simulink subsystem "WindGFMTurbineInertia23a"  (R2023a)
settings: Solver=VariableStepAuto  StartTime=0.0  StopTime=10.0  RelTol=1e-3
model mask{Kp=0, D=0, H=0, KqI=0, Vd_ref=0, frequency=0, x_vir=0, r_vir=0, Imax=0, Radius1=0, pitch1=0, cp1=0, TSR1=0, airDensity1=0, wt1=0, rt1=0, Inertia1=0, p1=0, psim1=0, Ld1=0, Lq1=0, Rs1=0, Kp_dc_sm=0, Ki_dc_sm=0, Kpd=0, Kid=0, Kpq=0, Kiq=0}
  mask prompts: Kp "VSM frequency droop"; D "VSM damping"; H "VSM Inertia"; KqI "VSM Reactive power droop"; Vd_ref "Volatge Reference d-axis"; frequency "Reference frequency"; x_vir "Virtual reactance"; r_vir "Virtual resistance"; Imax "Current limit"; Radius1 "Radius of Turbine"; pitch1 "Pitch Angle Vector"; cp1 "Power Coefficient Table"; TSR1 "Tip Speed Ratio"; airDensity1 "Air Density"; wt1 "Wind Velocity Threshold"; rt1 "Rotational Velocity Threshold"; Inertia1 "Turbine Inertia"; p1 "Number of Pole Pairs"; psim1 "PM Flux Linkage"; Ld1 "Stator D-axis inductance (H)"; Lq1 "Stator Q-axis inductance (H)"; Rs1 "Stator Resistance (Ohms)"; Kp_dc_sm "Prportional Gain of Dc-link Controller"; Ki_dc_sm "Integral Gain of DC-link Controller"; Kpd "D-axis proportional Gain"; Kid "D-axis integral Gain"; Kpq "q-axis proportional Gain"; Kiq "q-axis integral Gain"
undefined symbols (not defined in the file): alpha, base, DiscIntNeverNeededParam, Ld, Lq, mpptPower, mpptWindSpeed, p, psim, Rs, Ts, windController, windInverter, windTurbine
libraries: nesl_utility x14, ee_lib x9, fl_lib x7, slpidlib x5, eeTransforms x5, eeGeneralControl x2, simulink x2, eePowerMeasurement x1, eePmsmCurrentController x1
(part 1 of 2)
settings Model: Creator=rajarshd  LastModifiedBy=rajarshd
settings DebuggingCC: SubsystemReferenceDiagnosticForUnitTest=warning

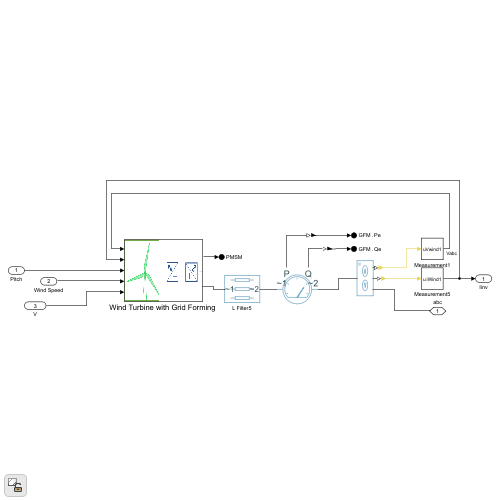
[thumbnail: Simulink's stored preview of the top-level diagram]
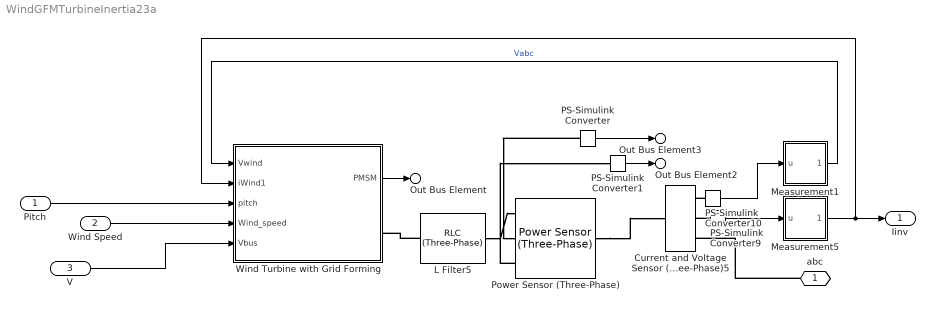
== system WindGFMTurbineInertia23a ==
  Pitch : Inport
  Wind Speed : Inport  Port=2
  V : Inport  Port=3
  Current and Voltage Sensor (Three-Phase)5 : ee_lib/Sensors & Transducers/Current and Voltage Sensor (Three-Phase)  vMeasurementType=ee.enum.vmeasurement.lg  outputUnit=ee.enum.unit.pu  SRated=base.mVA A*V  VRated=base.kV V  I_specify=off  I_priority=None  I=[0, 0, 0] A  I_nominal_specify=off  I_nominal_unit=A  I_nominal_value=1  V_specify=off  V_priority=None  V=[0, 0, 0] V  V_nominal_specify=off  V_nominal_unit=V  V_nominal_value=1
      settings: InternalSimscapePortConfiguration="{\"Bottom\":[],\"Left\":[{\"id\":\"N1\",\"label\":\"~1\",\"type\":\"foundation.electrical.three_phase\"}],\"Right\":[{\"id\":\"V_output\",\"label\":\"V\",\"type\":\"output\"},{\"id\":\"I_output\",\"label\":\"I\",\"type\":\"output\"},{\"id\":\"N2\",\"label\":\"~2\",\"type\":\"foundation.electrical.three_phase\"}],\"Top\":[]}"
  L Filter5 : ee_lib/Passive/RLC Assemblies/RLC (Three-Phase)  component_structure=ee.enum.rlc.structure.L  R=1e-3 Ohm  L=windInverter.l*1 H  C=1e-6 F  R_parasitic=0 Ohm  G_parasitic=0 1/Ohm  IL_specify=off  IL_priority=High  IL=[0, 0, 0] A  IL_nominal_specify=off  IL_nominal_unit=A  IL_nominal_value=1  VC_specify=off  VC_priority=High  VC=[0, 0, 0] V  VC_nominal_specify=off  VC_nominal_unit=V  VC_nominal_value=1
      settings: InternalSimscapePortConfiguration="{\"Bottom\":[],\"Left\":[{\"id\":\"N1\",\"label\":\"~1\",\"type\":\"foundation.electrical.three_phase\"}],\"Right\":[{\"id\":\"N2\",\"label\":\"~2\",\"type\":\"foundation.electrical.three_phase\"}],\"Top\":[]}"
  Measurement1 : Subsystem
  Measurement5 : Subsystem
  PS-Simulink Converter{,1,9..10} (4 alike) : nesl_utility/PS-Simulink Converter  PhysicalDomain=network_engine_domain  SubClassName=ps_output  LeftPortType=input  RightPortType=output  PseudoPeriodic=off  Frequencies=[]  VectorFormat=inherit  Unit=inherit  AffineConversion=off
  Power Sensor (Three-Phase) : ee_lib/Sensors & Transducers/Power Sensor (Three-Phase)  load_type=ee.enum.passive.type_balanced.balanced  f0=60 Hz  config=ee.enum.with_neutral.no  rho=1
      settings: InternalSimscapePortConfiguration="{\"Bottom\":[],\"Left\":[{\"id\":\"N1\",\"label\":\"~1\",\"type\":\"foundation.electrical.three_phase\"}],\"Right\":[{\"id\":\"N2\",\"label\":\"~2\",\"type\":\"foundation.electrical.three_phase\"}],\"Top\":[{\"id\":\"Pm\",\"label\":\"P\",\"type\":\"output\"},{\"id\":\"Qm\",\"label\":\"Q\",\"type\":\"output\"}]}"
  "Wind Turbine with Grid Forming " : Subsystem
      mask Display: image('T4wind.png'); % Use "Edit Image" on toolstrip to change.
  abc : PMIOPort  Side=Right
  Iinv : Outport
  Out Bus Element : Outport  Port=2  PortName=PMSM
  Out Bus Element2 : Outport  Port=3  PortName=GFM  Element=Qe
  Out Bus Element3 : Outport  Port=3  PortName=GFM  Element=Pe
  wires:
  V/1 -> "Wind Turbine with Grid Forming "/5(Vbus)
  Measurement1/1(Vwind1) -> "Wind Turbine with Grid Forming "/1(Vwind)  "Vabc"
  PS-Simulink Converter9/1 -> Measurement5/1(u)
  Measurement5/1(iWind1) -> "Wind Turbine with Grid Forming "/2(iWind1), Iinv/1
  PS-Simulink Converter10/1 -> Measurement1/1(u)
  Wind Speed/1 -> "Wind Turbine with Grid Forming "/4(Wind_speed)
  Pitch/1 -> "Wind Turbine with Grid Forming "/3(pitch)
  "Wind Turbine with Grid Forming "/1(PMSM) -> Out Bus Element/1
  PS-Simulink Converter/1 -> Out Bus Element3/1
  PS-Simulink Converter1/1 -> Out Bus Element2/1
  connections:
  L Filter5/LConn1 -- "Wind Turbine with Grid Forming "/RConn1
  PS-Simulink Converter9/LConn1 -- Current and Voltage Sensor (Three-Phase)5/RConn2
  PS-Simulink Converter10/LConn1 -- Current and Voltage Sensor (Three-Phase)5/RConn1
  abc/RConn1 -- Current and Voltage Sensor (Three-Phase)5/RConn3
  Power Sensor (Three-Phase)/RConn1 -- Current and Voltage Sensor (Three-Phase)5/LConn1
  PS-Simulink Converter/LConn1 -- Power Sensor (Three-Phase)/LConn2
  Power Sensor (Three-Phase)/LConn3 -- PS-Simulink Converter1/LConn1
  L Filter5/RConn1 -- Power Sensor (Three-Phase)/LConn1

== system WindGFMTurbineInertia23a/Measurement1 ==
  u : Inport
  Lead-Lag (Discrete or Continuous) : eeGeneralControl/Lead-Lag (Discrete or Continuous)  T1=0  T2=windController.tSensor  B=inf  A=-inf  init_option=Inherited from block input  x0=0  Ts=Ts
      settings: LibrarySourceBlock=|
      | ee_sl_lib/General Control/Lead-Lag
      | (Discrete or Continuous)
  Out Bus Element : Outport  PortName=Vwind1
  wires:
  u/1 -> Lead-Lag (Discrete or Continuous)/1
  Lead-Lag (Discrete or Continuous)/1 -> Out Bus Element/1

== system WindGFMTurbineInertia23a/Measurement5 ==
  u : Inport
  Lead-Lag (Discrete or Continuous) : eeGeneralControl/Lead-Lag (Discrete or Continuous)  T1=0  T2=windController.tSensor  B=inf  A=-inf  init_option=Inherited from block input  x0=0  Ts=Ts
      settings: LibrarySourceBlock=|
      | ee_sl_lib/General Control/Lead-Lag
      | (Discrete or Continuous)
  Out Bus Element : Outport  PortName=iWind1  Element=1
  wires:
  u/1 -> Lead-Lag (Discrete or Continuous)/1
  Lead-Lag (Discrete or Continuous)/1 -> Out Bus Element/1

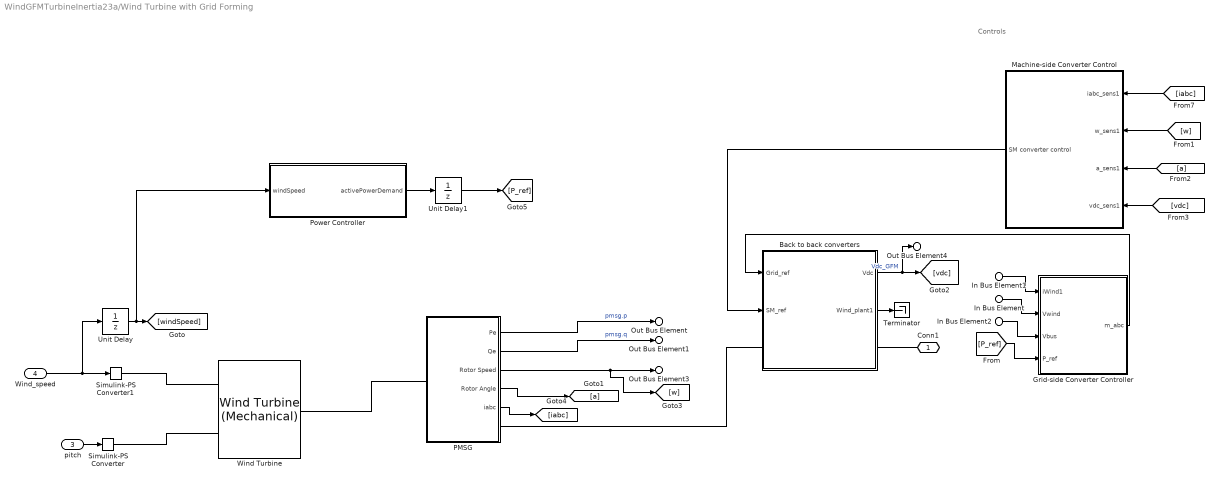
== system WindGFMTurbineInertia23a/Wind Turbine with Grid Forming  ==
  note: Controls
  In Bus Element : Inport  PortName=Vwind
  In Bus Element1 : Inport  Port=2  PortName=iWind1
  pitch : Inport  Port=3
  Wind_speed : Inport  Port=4
  In Bus Element2 : Inport  Port=5  PortName=Vbus
  " Grid-side Converter Controller" : Subsystem
  Back to back converters : Subsystem
  Machine-side Converter Control : Subsystem
  PMSG : Subsystem
  Power Controller : Subsystem
  Simulink-PS Converter : nesl_utility/Simulink-PS Converter  PhysicalDomain=network_engine_domain  SubClassName=ps_input  LeftPortType=input  RightPortType=output  PseudoPeriodic=off  Frequencies=[]  NoiseDistribution=none  NoiseParameters=[]  Unit=1  AffineConversion=off  FilteringAndDerivatives=provide  SimscapeFilterOrder=1  InputFilterTimeConstant=0.001  UdotUserProvided=0
  Simulink-PS Converter1 : nesl_utility/Simulink-PS Converter  PhysicalDomain=network_engine_domain  SubClassName=ps_input  LeftPortType=input  RightPortType=output  PseudoPeriodic=off  Frequencies=[]  NoiseDistribution=none  NoiseParameters=[]  Unit=1  AffineConversion=off  FilteringAndDerivatives=provide  SimscapeFilterOrder=1  InputFilterTimeConstant=0.001  UdotUserProvided=0
  Terminator : Terminator
  Unit Delay : UnitDelay  SampleTime=-1  HasFrameUpgradeWarning=on
  Unit Delay1 : UnitDelay  SampleTime=-1  HasFrameUpgradeWarning=on
  "Wind Turbine " : ee_lib/Electromechanical/Wind Turbine (Mechanical)  R_rotor=Radius1 m  pitch_TLU=pitch1 deg  lambda_TLU=TSR1  Cp_TLU=cp1  v_thr=wt1 m/s  w_thr=rt1 rad/s  rho_air=airDensity1 kg/m^3  includeInertia=true  J=Inertia1 kg*m^2  lam=1 N*m*s/rad  w_specify=on  w_priority=Low  w=2.26*2 rad/s  w_nominal_specify=off  w_nominal_unit=rad/s  w_nominal_value=1  t_specify=off  t_priority=None  t=0 N*m  t_nominal_specify=off  t_nominal_unit=N*m  t_nominal_value=1  Torque_specify=off  Torque_priority=None  Torque=0 N*m  Torque_nominal_specify=off  Torque_nominal_unit=N*m  Torque_nominal_value=1
      settings: InternalSimscapePortConfiguration="{\"Bottom\":[],\"Left\":[{\"id\":\"vWind\",\"label\":\"V\",\"type\":\"input\"},{\"id\":\"pitch\",\"label\":\"β\",\"type\":\"input\"}],\"Right\":[{\"id\":\"R\",\"label\":\"R\",\"type\":\"foundation.mechanical.rotational.rotational\"}],\"Top\":[]}"
  Conn1 : PMIOPort  Side=Right
  Out Bus Element : Outport  PortName=PMSM  Element=P_GFM
  Out Bus Element1 : Outport  PortName=PMSM  Element=Q_GFM
  Out Bus Element3 : Outport  PortName=PMSM  Element=w_speed_GFM
  Out Bus Element4 : Outport  PortName=PMSM  Element=Vdc_GFM
  wires:
  [iabc] -> Machine-side Converter Control/1(iabc_sens1)
  [w] -> Machine-side Converter Control/2(w_sens1)
  [a] -> Machine-side Converter Control/3(a_sens1)
  [vdc] -> Machine-side Converter Control/4(vdc_sens1)
  PMSG/3(Rotor Speed) -> [w], Out Bus Element3/1
  PMSG/2(Qe) -> Out Bus Element1/1  "pmsg.q"
  In Bus Element1/1 -> " Grid-side Converter Controller"/1(iWind1)
  Wind_speed/1 -> Simulink-PS Converter1/1, Unit Delay/1
  pitch/1 -> Simulink-PS Converter/1
  PMSG/5(iabc) -> [iabc]
  Back to back converters/1(Vdc) -> Out Bus Element4/1, [vdc]  "Vdc_GFM"
  PMSG/4(Rotor Angle) -> [a]
  PMSG/1(Pe) -> Out Bus Element/1  "pmsg.p"
  Unit Delay/1 -> Power Controller/1(windSpeed), [windSpeed]
  In Bus Element/1 -> " Grid-side Converter Controller"/2(Vwind)
  In Bus Element2/1 -> " Grid-side Converter Controller"/3(Vbus)
  Unit Delay1/1 -> [P_ref]
  Power Controller/1(activePowerDemand) -> Unit Delay1/1
  [P_ref] -> " Grid-side Converter Controller"/4(P_ref)
  Back to back converters/2(Wind_plant1) -> Terminator/1
  Machine-side Converter Control/1(SM converter control) -> Back to back converters/2(SM_ref)
  " Grid-side Converter Controller"/1(m_abc) -> Back to back converters/1(Grid_ref)
  connections:
  PMSG/RConn1 -- Back to back converters/LConn1
  "Wind Turbine "/RConn1 -- PMSG/LConn1
  "Wind Turbine "/LConn2 -- Simulink-PS Converter/RConn1
  "Wind Turbine "/LConn1 -- Simulink-PS Converter1/RConn1
  Conn1/RConn1 -- Back to back converters/RConn1

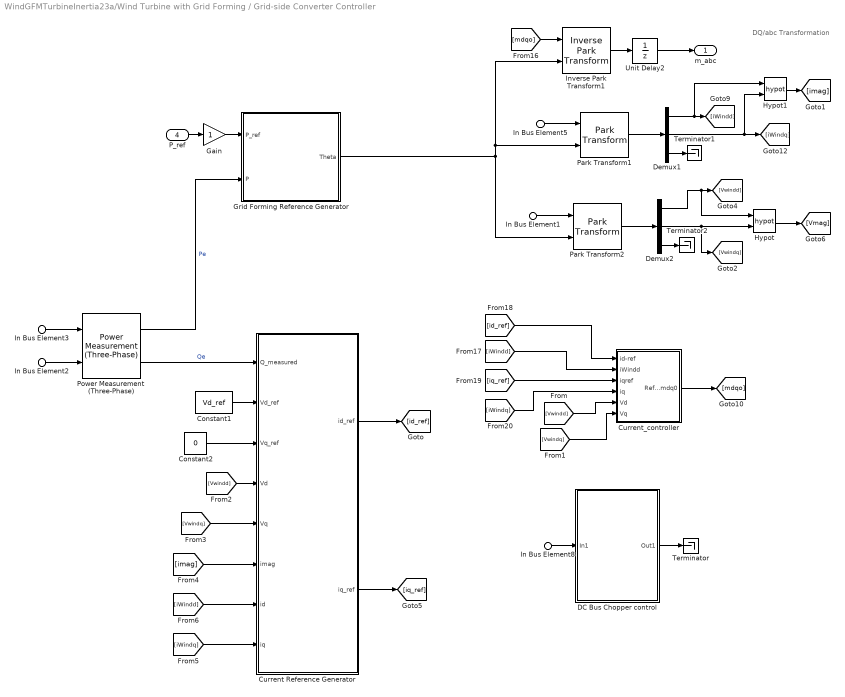
== system WindGFMTurbineInertia23a/Wind Turbine with Grid Forming / Grid-side Converter Controller ==
  note: DQ/abc Transformation
  In Bus Element5 : Inport  PortName=iWind1
  In Bus Element2 : Inport  PortName=iWind1
  In Bus Element1 : Inport  Port=2  PortName=Vwind
  In Bus Element3 : Inport  Port=2  PortName=Vwind
  In Bus Element8 : Inport  Port=3  PortName=Vbus  Element=Vmag
  P_ref : Inport  Port=4
  Constant1 : Constant  Value=Vd_ref
  Constant2 : Constant  Value=0
  Current Reference Generator : Subsystem
  Current_controller : Subsystem
  "DC Bus Chopper control " : Subsystem
  Demux1 : Demux  Outputs=3
  Demux2 : Demux  Outputs=3
  Gain : Gain
  Grid Forming Reference Generator : Subsystem
  Hypot : Math  Operator=hypot  SignedPower=on  RndMeth=Zero
  Hypot1 : Math  Operator=hypot
  Inverse Park Transform1 : eeTransforms/Inverse Park Transform  AxisAlignment=Q-axis  PowerInvariant=off
  Park Transform1 : eeTransforms/Park Transform  AxisAlignment=Q-axis  PowerInvariant=off
  Park Transform2 : eeTransforms/Park Transform  AxisAlignment=Q-axis  PowerInvariant=off
  Power Measurement (Three-Phase) : eePowerMeasurement/Power Measurement (Three-Phase)  LabelModeActiveChoice=Discrete  F=60  K=[1]  Seq=Positive  Ts=Ts
  Terminator : Terminator
  Terminator1 : Terminator
  Terminator2 : Terminator
  Unit Delay2 : UnitDelay  SampleTime=Ts  HasFrameUpgradeWarning=on
  m_abc : Outport
  wires:
  Gain/1 -> Grid Forming Reference Generator/1(P_ref)
  "DC Bus Chopper control "/1(Out1) -> Terminator/1
  In Bus Element8/1 -> "DC Bus Chopper control "/1(In1)
  [iWindq] -> Current Reference Generator/8(iq)
  [iWindd] -> Current Reference Generator/7(id)
  [imag] -> Current Reference Generator/6(imag)
  Hypot1/1 -> [imag]
  [Vwindq] -> Current Reference Generator/5(Vq)
  [Vwindd] -> Current Reference Generator/4(Vd)
  Constant2/1 -> Current Reference Generator/3(Vq_ref)
  Constant1/1 -> Current Reference Generator/2(Vd_ref)
  Power Measurement (Three-Phase)/2 -> Current Reference Generator/1(Q_measured)  "Qe"
  Power Measurement (Three-Phase)/1 -> Grid Forming Reference Generator/2(P)  "Pe"
  Current Reference Generator/2(iq_ref) -> [iq_ref]
  Current Reference Generator/1(id_ref) -> [id_ref]
  Grid Forming Reference Generator/1(Theta) -> Park Transform2/2, Park Transform1/2, Inverse Park Transform1/2
  In Bus Element3/1 -> Power Measurement (Three-Phase)/1
  In Bus Element2/1 -> Power Measurement (Three-Phase)/2
  Hypot/1 -> [Vmag]
  [Vwindq] -> Current_controller/6(Vq)
  [Vwindd] -> Current_controller/5(Vd)
  In Bus Element1/1 -> Park Transform2/1
  Demux2/2 -> [Vwindq], Hypot/2
  Demux2/3 -> Terminator2/1
  Demux2/1 -> [Vwindd], Hypot/1
  Park Transform2/1 -> Demux2/1
  Current_controller/1(Refrence_mdq0) -> [mdqo]
  Inverse Park Transform1/1 -> Unit Delay2/1
  Demux1/2 -> [iWindq], Hypot1/2
  Unit Delay2/1 -> m_abc/1
  Demux1/1 -> [iWindd], Hypot1/1
  Demux1/3 -> Terminator1/1
  [mdqo] -> Inverse Park Transform1/1
  Park Transform1/1 -> Demux1/1
  [id_ref] -> Current_controller/1(id-ref)
  [iq_ref] -> Current_controller/3(iqref)
  [iWindq] -> Current_controller/4(iq)
  [iWindd] -> Current_controller/2(iWindd)
  In Bus Element5/1 -> Park Transform1/1
  P_ref/1 -> Gain/1

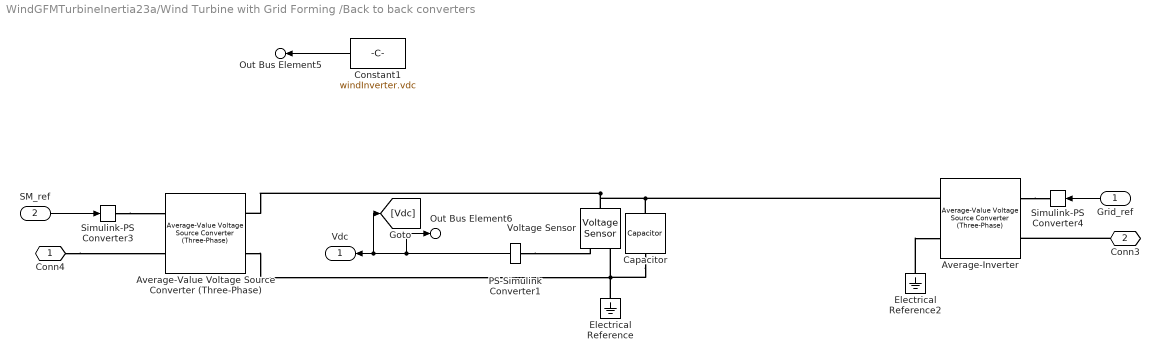
== system WindGFMTurbineInertia23a/Wind Turbine with Grid Forming /Back to back converters ==
  Grid_ref : Inport
  SM_ref : Inport  Port=2
  Average-Inverter : ee_lib/Semiconductors & Converters/Converters/Average-Value Voltage Source Converter (Three-Phase)  port_option=ee.enum.threePhasePort.composite  frequency_option=ee.enum.converters.frequency.variable  FRated=60 Hz  losses_parameterization=ee.enum.converters.losses.fixed  Pfixed=1 W  ks=0.01  kc1=1.7 V  kc2=0.01 Ohm  Ploss_vect=[100, 800, 1870, 3250, 4900] W  Irms_vect=[10, 100, 200, 300, 400] A  Vdc_nom=300 V  thermal_mass=30000 J/K  temperature_specify=off  temperature_priority=High  temperature=298.15 K  temperature_nominal_specify=off  temperature_nominal_unit=K  temperature_nominal_value=1
      settings: InternalSimscapePortConfiguration="{\"Bottom\":[],\"Left\":[{\"id\":\"ModWave\",\"label\":\"ModWave\",\"type\":\"input\"},{\"id\":\"N\",\"label\":\"~\",\"type\":\"foundation.electrical.three_phase\"}],\"Right\":[{\"id\":\"p\",\"label\":\"+\",\"type\":\"foundation.electrical.electrical\"},{\"id\":\"n\",\"label\":\"-\",\"type\":\"foundation.electrical.electrical\"}],\"Top\":[]}"
  Average-Value Voltage Source Converter (Three-Phase) : ee_lib/Semiconductors & Converters/Converters/Average-Value Voltage Source Converter (Three-Phase)  port_option=ee.enum.threePhasePort.composite  frequency_option=ee.enum.converters.frequency.variable  FRated=60 Hz  losses_parameterization=ee.enum.converters.losses.fixed  Pfixed=1 W  ks=0.01  kc1=1.7 V  kc2=0.01 Ohm  Ploss_vect=[100, 800, 1870, 3250, 4900] W  Irms_vect=[10, 100, 200, 300, 400] A  Vdc_nom=300 V  thermal_mass=30000 J/K  temperature_specify=off  temperature_priority=High  temperature=298.15 K  temperature_nominal_specify=off  temperature_nominal_unit=K  temperature_nominal_value=1
      settings: InternalSimscapePortConfiguration="{\"Bottom\":[],\"Left\":[{\"id\":\"ModWave\",\"label\":\"ModWave\",\"type\":\"input\"},{\"id\":\"N\",\"label\":\"~\",\"type\":\"foundation.electrical.three_phase\"}],\"Right\":[{\"id\":\"p\",\"label\":\"+\",\"type\":\"foundation.electrical.electrical\"},{\"id\":\"n\",\"label\":\"-\",\"type\":\"foundation.electrical.electrical\"}],\"Top\":[]}"
  Capacitor : fl_lib/Electrical/Electrical Elements/Capacitor  c=windInverter.c*2.5 F  r=0.001 Ohm  g=0 1/Ohm  i_specify=off  i_priority=None  i=0 A  i_nominal_specify=off  i_nominal_unit=A  i_nominal_value=1  v_specify=off  v_priority=None  v=0 V  v_nominal_specify=off  v_nominal_unit=V  v_nominal_value=1  vc_specify=on  vc_priority=None  vc=windInverter.vdc V  vc_nominal_specify=off  vc_nominal_unit=V  vc_nominal_value=1
  Constant1 : Constant  Value=windInverter.vdc  SampleTime=Ts
  Electrical Reference : fl_lib/Electrical/Electrical Elements/Electrical Reference
  Electrical Reference2 : fl_lib/Electrical/Electrical Elements/Electrical Reference
  PS-Simulink Converter1 : nesl_utility/PS-Simulink Converter  PhysicalDomain=network_engine_domain  SubClassName=ps_output  LeftPortType=input  RightPortType=output  PseudoPeriodic=off  Frequencies=[]  VectorFormat=inherit  Unit=V  AffineConversion=off
  Simulink-PS Converter3 : nesl_utility/Simulink-PS Converter  PhysicalDomain=network_engine_domain  SubClassName=ps_input  LeftPortType=input  RightPortType=output  PseudoPeriodic=off  Frequencies=[]  NoiseDistribution=none  NoiseParameters=[]  Unit=1  AffineConversion=off  FilteringAndDerivatives=provide  SimscapeFilterOrder=1  InputFilterTimeConstant=0.001  UdotUserProvided=0
  Simulink-PS Converter4 : nesl_utility/Simulink-PS Converter  PhysicalDomain=network_engine_domain  SubClassName=ps_input  LeftPortType=input  RightPortType=output  PseudoPeriodic=off  Frequencies=[]  NoiseDistribution=none  NoiseParameters=[]  Unit=1  AffineConversion=off  FilteringAndDerivatives=provide  SimscapeFilterOrder=1  InputFilterTimeConstant=0.001  UdotUserProvided=0
  Voltage Sensor : fl_lib/Electrical/Electrical Sensors/Voltage Sensor
  Conn4 : PMIOPort  Side=Left
  Conn3 : PMIOPort  Port=2  Side=Right
  Vdc : Outport
  Out Bus Element6 : Outport  Port=2  PortName=Wind_plant1  Element=Vdc_measured
  Out Bus Element5 : Outport  Port=2  PortName=Wind_plant1  Element=windInverter.vdc
  wires:
  PS-Simulink Converter1/1 -> Out Bus Element6/1, Vdc/1, [Vdc]
  Grid_ref/1 -> Simulink-PS Converter4/1
  SM_ref/1 -> Simulink-PS Converter3/1
  Constant1/1 -> Out Bus Element5/1
  connections:
  Capacitor/LConn1 -- Voltage Sensor/LConn1 -- Average-Value Voltage Source Converter (Three-Phase)/RConn1 -- Average-Inverter/RConn1
  Capacitor/RConn1 -- Voltage Sensor/RConn2 -- Average-Value Voltage Source Converter (Three-Phase)/RConn2 -- Electrical Reference/LConn1
  PS-Simulink Converter1/LConn1 -- Voltage Sensor/RConn1
  Electrical Reference2/LConn1 -- Average-Inverter/RConn2
  Conn4/RConn1 -- Average-Value Voltage Source Converter (Three-Phase)/LConn2
  Average-Inverter/LConn1 -- Simulink-PS Converter4/RConn1
  Simulink-PS Converter3/RConn1 -- Average-Value Voltage Source Converter (Three-Phase)/LConn1
  Conn3/RConn1 -- Average-Inverter/LConn2

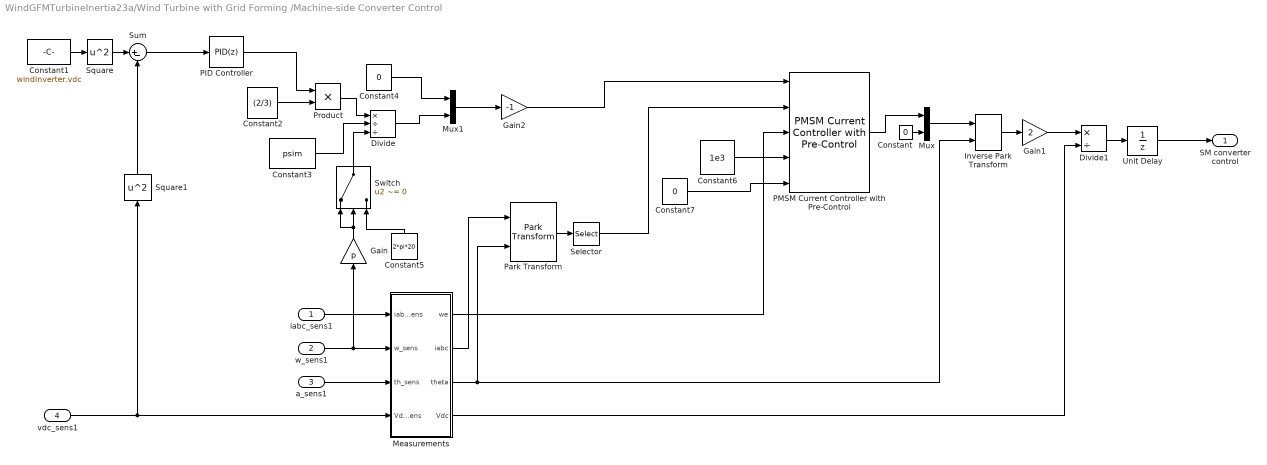
== system WindGFMTurbineInertia23a/Wind Turbine with Grid Forming /Machine-side Converter Control ==
  iabc_sens1 : Inport
  w_sens1 : Inport  Port=2
  a_sens1 : Inport  Port=3
  vdc_sens1 : Inport  Port=4
  Constant : Constant  Value=0  SampleTime=-1
  Constant1 : Constant  Value=windInverter.vdc
  Constant2 : Constant  Value=(2/3)
  Constant3 : Constant  Value=psim
  Constant4 : Constant  Value=0
  Constant5 : Constant  Value=2*pi*20
  Constant6 : Constant  Value=1e3  VectorParams1D=off  SampleTime=-1
  Constant7 : Constant  Value=0
  Divide : Product  Inputs=*//
  Divide1 : Product  Inputs=*/
  Gain : Gain  Gain=p
  Gain1 : Gain  Gain=2
  Gain2 : Gain  Gain=-1
  Inverse Park Transform : eeTransforms/Inverse Park Transform  AxisAlignment=Q-axis  PowerInvariant=off
  Measurements : Subsystem
  Mux : Mux  Inputs=2
  Mux1 : Mux  Inputs=2
  PID Controller : slpidlib/PID Controller  Controller=PID  Form=Parallel  TimeDomain=Discrete-time  UseExternalTs=off  SampleTime=-1  IntegratorMethod=Forward Euler  FilterMethod=Forward Euler  ControllerParametersSource=internal  P=Kp_dc_sm  I=Ki_dc_sm  UseKiTs=off  D=0  N=100  UseFilter=on  TunerSelectOption=Transfer Function Based (PID Tuner App)  InitialConditionSource=internal  InitialConditionForIntegrator=0  InitialConditionForFilter=0  DifferentiatorICPrevScaledInput=0  ExternalReset=none  TrackingMode=off  Kt=1  LimitOutput=off  SatLimitsSource=internal  UpperSaturationLimit=10e6  LowerSaturationLimit=-10e6  LinearizeAsGain=on  AntiWindupMode=none  Kb=1  LimitIntegrator=off  UpperIntegratorSaturationLimit=inf  LowerIntegratorSaturationLimit=-inf  POutMin=[]  POutMax=[]  IOutMin=[]  IOutMax=[]  DOutMin=[]  DOutMax=[]  NOutMin=[]  NOutMax=[]  SumOutMin=[]  SumOutMax=[]  SaturationOutMin=[]  SaturationOutMax=[]  PParamMin=[]  PParamMax=[]  IParamMin=[]  IParamMax=[]  DParamMin=[]  DParamMax=[]  NParamMin=[]  NParamMax=[]  KbParamMin=[]  KbParamMax=[]  KtParamMin=[]  KtParamMax=[]  KbOutMin=[]  KbOutMax=[]  KtOutMin=[]  KtOutMax=[]  IntegratorOutMin=[]  IntegratorOutMax=[]  FilterOutMin=[]  FilterOutMax=[]  SumI1OutMin=[]  SumI1OutMax=[]  SumI2OutMin=[]  SumI2OutMax=[]  SumI3OutMin=[]  SumI3OutMax=[]  SumI4OutMin=[]  SumI4OutMax=[]  SumDOutMin=[]  SumDOutMax=[]  DifferentiatorOutMin=[]  DifferentiatorOutMax=[]  FilterDiffOutCoefMin=[]  FilterDiffOutCoefMax=[]  ReciprocalOutMin=[]  ReciprocalOutMax=[]  SumDenOutMin=[]  SumDenOutMax=[]  SumNumOutMin=[]  SumNumOutMax=[]  DivideOutMin=[]  DivideOutMax=[]  UdiffTsProdOutMin=[]  UdiffTsProdOutMax=[]  NTsProdOutMin=[]  NTsProdOutMax=[]  UintegralTsProdOutMin=[]  UintegralTsProdOutMax=[]  UngainTsProdOutMin=[]  UngainTsProdOutMax=[]  ClampingZeroOutDataTypeStr=Inherit: Inherit via back propagation  ClampingZeroOutMin=[]  ClampingZeroOutMax=[]  FilterDenConstantOutDataTypeStr=Inherit: Inherit via back propagation  FilterDenConstantOutMin=[]  FilterDenConstantOutMax=[]  PCopyOutDataTypeStr=Inherit: Inherit via back propagation  PCopyOutMin=[]  PCopyOutMax=[]  NCopyOutDataTypeStr=Inherit: Inherit via back propagation  NCopyOutMin=[]  NCopyOutMax=[]  IntegratorContinuousStateAttributes=''  IntegratorStateMustResolveToSignalObject=off  IntegratorRTWStateStorageClass=Auto  FilterContinuousStateAttributes=''  FilterStateMustResolveToSignalObject=off  FilterRTWStateStorageClass=Auto  ParallelPVariant=InternalParameters  IdealPVariant=Disabled  IVariant=InternalParameters  DVariant=InternalParameters  IntegratorVariant=Discrete  SatVariant=Disabled  AWVariant=Passthrough  PCopyVariant=Disabled  TRVariant=Disabled  FdbkBlocksVariant=Forward  IdealPFdbkVariant=Disabled  SatFdbkVariant=Disabled  DerivativeFilterVariant=ForwardEulerFilter  NVariant=InternalParameters  NCopyVariant=Disabled  FilterICVariant=InternalICsFilter  IntegratorICVariant=InternalICs  ExternalResetVariant=Disabled  TRSumVariant=Passthrough  SumFdbkVariant=Disabled  SumVariant=Sum_PID  TsampFilterVariant=InternalTs  TsampNgainVariant=Passthrough  TsampIntegralVariant=Disabled_SignalSpec  ExternalSaturationOutDataTypeStr=Inherit: Same as second input
  PMSM Current Controller with Pre-Control : eePmsmCurrentController/PMSM Current Controller with Pre-Control  Kp_id=Kpd %Ld*alpha  Ki_id=Kid %Rs*alpha  Kaw_id=0  Kp_iq=Kpq %Lq*alpha  Ki_iq=Kiq %Rs*alpha  Kaw_iq=0  Ts=-1  Tsd=0.001  AxisPrio=Q-axis  ActZC=off  ActFF=on  idVect=[-1, 0, 1]  iqVect=[-2000, 0, 2000]  LdMatrix=Ld* ones(3, 3)  LqMatrix=Lq* ones(3, 3)  psimMatrix=psim * ones(3, 3)
      settings: LibrarySourceBlock=|
      | ee_sl_lib/PMSM Control/PMSM Current Controller
      | with Pre-Control
  Park Transform : eeTransforms/Park Transform  AxisAlignment=Q-axis  PowerInvariant=off
  Product : Product
  Selector : Selector  InputPortWidth=3  IndexOptions=Index vector (dialog)  Indices=[1 2]  OutputSizes=1
  Square : Math  Operator=square
  Square1 : Math  Operator=square
  Sum : Sum  Inputs=|+-
  Switch : Switch  Criteria=u2 ~= 0  SaturateOnIntegerOverflow=off  InputSameDT=off
  Unit Delay : UnitDelay  SampleTime=-1  HasFrameUpgradeWarning=on
  SM converter control : Outport  VectorParamsAs1DForOutWhenUnconnected=off
  wires:
  Square1/1 -> Sum/2
  Square/1 -> Sum/1
  Constant1/1 -> Square/1
  Unit Delay/1 -> SM converter control/1
  PMSM Current Controller with Pre-Control/1 -> Mux/1
  Constant4/1 -> Mux1/1
  Constant3/1 -> Divide/2
  a_sens1/1 -> Measurements/3(th_sens)
  Constant5/1 -> Switch/3
  Product/1 -> Divide/1
  Gain2/1 -> PMSM Current Controller with Pre-Control/1
  Mux1/1 -> Gain2/1
  Constant7/1 -> PMSM Current Controller with Pre-Control/5
  Measurements/3(theta) -> Park Transform/2, Inverse Park Transform/2
  vdc_sens1/1 -> Measurements/4(Vdc_sens), Square1/1
  Measurements/1(we) -> PMSM Current Controller with Pre-Control/3
  Park Transform/1 -> Selector/1
  iabc_sens1/1 -> Measurements/1(iabc_sens)
  Constant6/1 -> PMSM Current Controller with Pre-Control/4
  Divide1/1 -> Unit Delay/1
  Selector/1 -> PMSM Current Controller with Pre-Control/2
  Inverse Park Transform/1 -> Gain1/1
  Constant2/1 -> Product/2
  Mux/1 -> Inverse Park Transform/1
  Measurements/2(iabc) -> Park Transform/1
  Gain/1 -> Switch/1, Switch/2
  Constant/1 -> Mux/2
  Switch/1 -> Divide/3
  Gain1/1 -> Divide1/1
  w_sens1/1 -> Gain/1, Measurements/2(w_sens)
  Divide/1 -> Mux1/2
  PID Controller/1 -> Product/1
  Measurements/4(Vdc) -> Divide1/2
  Sum/1 -> PID Controller/1

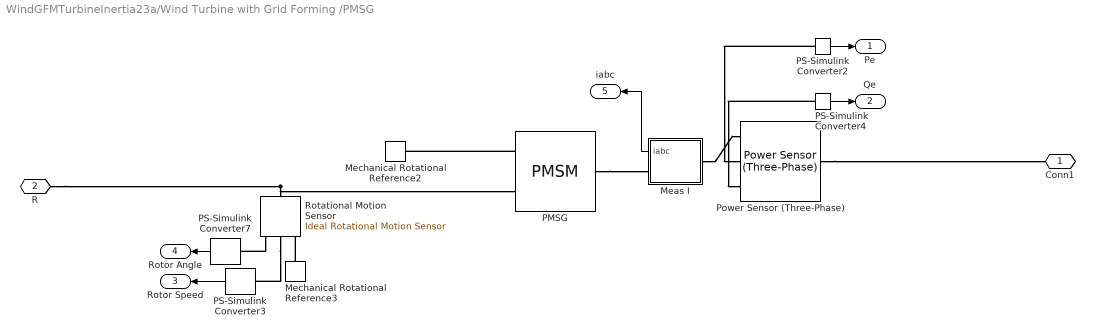
== system WindGFMTurbineInertia23a/Wind Turbine with Grid Forming /PMSG ==
  Meas I : Subsystem
  Mechanical Rotational Reference2 : fl_lib/Mechanical/Rotational Elements/Mechanical Rotational Reference
  Mechanical Rotational Reference3 : fl_lib/Mechanical/Rotational Elements/Mechanical Rotational Reference
  PMSG : ee_lib/Electromechanical/Permanent Magnet/PMSM  port_option=ee.enum.threePhasePort.composite  winding_type=ee.enum.statorconnection.wye  machine_param=ee.enum.pmsm.parameterization.constant  nPolePairs=p1  pmflux_param=ee.enum.pmflux.fluxlinkage  pm_flux_linkage=psim1 Wb  torque_constant=0.18 N*m/A  back_emf_constant=0.18 V*s/rad  stator_param=ee.enum.statorparam.LdLqL0  Ld=Ld1 H  Lq=Lq1 H  idVec=[-200, 0, 200] A  iqVec=[-200, 0, 200] A  LdMatrix=0.0002 * ones(3, 3) H  LqMatrix=0.0002 * ones(3, 3) H  PmMatrix=0.1 * ones(3, 3) Wb  ktMatrix=0.18 * ones(3, 3) N*m/A  keMatrix=0.18 * ones(3, 3) V*s/rad  L0=0.00016 H  Ls=0.0002 H  Lm=-0.00002 H  Ms=0.00002 H  Rs=Rs1 Ohm  zero_sequence=ee.enum.park.zerosequence.exclude  axes_param=ee.enum.rotorangle.qaxis  loss_param=ee.enum.ironloss.none  losses_oc=[0, 0, 0] W  losses_sc=[0, 0, 0] W  f_losses=60 Hz  Isc_losses=95 A  J=200 kg*m^2  lam=0 N*m*s/rad  i_d_specify=off  i_d_priority=None  i_d=0 A  i_d_nominal_specify=off  i_d_nominal_unit=A  i_d_nominal_value=1  i_q_specify=off  i_q_priority=None  i_q=0 A  i_q_nominal_specify=off  i_q_nominal_unit=A  i_q_nominal_value=1  torque_specify=off  torque_priority=None  torque=0 N*m  torque_nominal_specify=off  torque_nominal_unit=N*m  torque_nominal_value=1  angular_velocity_specify=on  angular_velocity_priority=High  angular_velocity=6 rad/s  angular_velocity_nominal_specify=off  angular_velocity_nominal_unit=rpm  angular_velocity_nominal_value=1  angular_position_specify=off  angular_position_priority=High  angular_position=0 deg  angular_position_nominal_specify=off  angular_position_nominal_unit=deg  angular_position_nominal_value=1  alpha=3.93e-3 1/K  alpha_flux=-0.001 1/K  Tmeas=298.15 K  stator_thermal_mass=100 J/K  rotor_thermal_mass=200 J/K  Rm_percent_rotor=90  Rd_percent_rotor=30  temperatureA_specify=off  temperatureA_priority=High  temperatureA=25 degC  temperatureA_nominal_specify=off  temperatureA_nominal_unit=degC  temperatureA_nominal_value=1  temperatureB_specify=off  temperatureB_priority=High  temperatureB=25 degC  temperatureB_nominal_specify=off  temperatureB_nominal_unit=degC  temperatureB_nominal_value=1  temperatureC_specify=off  temperatureC_priority=High  temperatureC=25 degC  temperatureC_nominal_specify=off  temperatureC_nominal_unit=degC  temperatureC_nominal_value=1  temperatureR_specify=off  temperatureR_priority=High  temperatureR=25 degC  temperatureR_nominal_specify=off  temperatureR_nominal_unit=degC  temperatureR_nominal_value=1
      settings: InternalSimscapePortConfiguration="{\"Bottom\":[],\"Left\":[{\"id\":\"N\",\"label\":\"~\",\"type\":\"foundation.electrical.three_phase\"}],\"Right\":[{\"id\":\"R\",\"label\":\"R\",\"type\":\"foundation.mechanical.rotational.rotational\"},{\"id\":\"C\",\"label\":\"C\",\"type\":\"foundation.mechanical.rotational.rotational\"}],\"Top\":[]}"
  PS-Simulink Converter2 : nesl_utility/PS-Simulink Converter  PhysicalDomain=network_engine_domain  SubClassName=ps_output  LeftPortType=input  RightPortType=output  PseudoPeriodic=off  Frequencies=[]  VectorFormat=inherit  Unit=inherit  AffineConversion=off
  PS-Simulink Converter3 : nesl_utility/PS-Simulink Converter  PhysicalDomain=network_engine_domain  SubClassName=ps_output  LeftPortType=input  RightPortType=output  PseudoPeriodic=off  Frequencies=[]  VectorFormat=inherit  Unit=rad/s  AffineConversion=off
  PS-Simulink Converter4 : nesl_utility/PS-Simulink Converter  PhysicalDomain=network_engine_domain  SubClassName=ps_output  LeftPortType=input  RightPortType=output  PseudoPeriodic=off  Frequencies=[]  VectorFormat=inherit  Unit=inherit  AffineConversion=off
  PS-Simulink Converter7 : nesl_utility/PS-Simulink Converter  PhysicalDomain=network_engine_domain  SubClassName=ps_output  LeftPortType=input  RightPortType=output  PseudoPeriodic=off  Frequencies=[]  VectorFormat=inherit  Unit=rad  AffineConversion=off
  Power Sensor (Three-Phase) : ee_lib/Sensors & Transducers/Power Sensor (Three-Phase)  load_type=ee.enum.passive.type_balanced.balanced  f0=60 Hz  config=ee.enum.with_neutral.no  rho=1
      settings: InternalSimscapePortConfiguration="{\"Bottom\":[],\"Left\":[{\"id\":\"N1\",\"label\":\"~1\",\"type\":\"foundation.electrical.three_phase\"}],\"Right\":[{\"id\":\"N2\",\"label\":\"~2\",\"type\":\"foundation.electrical.three_phase\"}],\"Top\":[{\"id\":\"Pm\",\"label\":\"P\",\"type\":\"output\"},{\"id\":\"Qm\",\"label\":\"Q\",\"type\":\"output\"}]}"
  Rotational Motion Sensor : fl_lib/Mechanical/Mechanical Sensors/Ideal Rotational Motion Sensor  reference=foundation.enum.MeasurementReference.difference  acceleration_port=false  velocity_port=true  position_port=true  wrap_angle=simscape.enum.onoff.off  offset=0 deg
  Conn1 : PMIOPort  Side=Right
  R : PMIOPort  Port=2  Side=Left
  Pe : Outport
  Qe : Outport  Port=2
  Rotor Speed : Outport  Port=3
  Rotor Angle : Outport  Port=4
  iabc : Outport  Port=5
  wires:
  Meas I/1(iabc) -> iabc/1
  PS-Simulink Converter7/1 -> Rotor Angle/1
  PS-Simulink Converter2/1 -> Pe/1
  PS-Simulink Converter4/1 -> Qe/1
  PS-Simulink Converter3/1 -> Rotor Speed/1
  connections:
  PMSG/RConn2 -- Mechanical Rotational Reference2/LConn1
  Rotational Motion Sensor/RConn2 -- PS-Simulink Converter3/LConn1
  Rotational Motion Sensor/RConn3 -- PS-Simulink Converter7/LConn1
  R/RConn1 -- PMSG/RConn1 -- Rotational Motion Sensor/LConn1
  Mechanical Rotational Reference3/LConn1 -- Rotational Motion Sensor/RConn1
  PS-Simulink Converter4/LConn1 -- Power Sensor (Three-Phase)/LConn3
  PS-Simulink Converter2/LConn1 -- Power Sensor (Three-Phase)/LConn2
  Power Sensor (Three-Phase)/RConn1 -- Conn1/RConn1
  Meas I/LConn1 -- Power Sensor (Three-Phase)/LConn1
  PMSG/LConn1 -- Meas I/RConn1

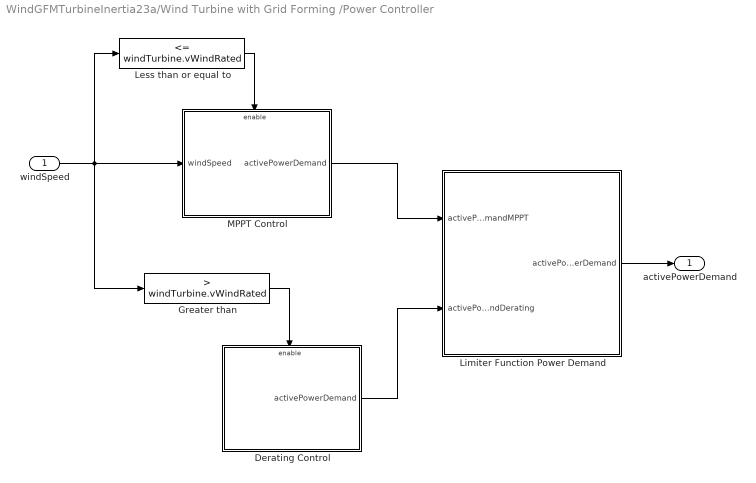
== system WindGFMTurbineInertia23a/Wind Turbine with Grid Forming /Power Controller ==
  windSpeed : Inport
  Derating Control : Subsystem
  Greater than : simulink/Logic and Bit Operations/Compare To Constant  relop=>  const=windTurbine.vWindRated  OutDataTypeStr=boolean
  Less than or equal to : simulink/Logic and Bit Operations/Compare To Constant  relop=<=  const=windTurbine.vWindRated  OutDataTypeStr=boolean
  Limiter Function Power Demand : Subsystem
  MPPT Control : Subsystem
  activePowerDemand : Outport
  wires:
  windSpeed/1 -> Greater than/1, Less than or equal to/1, MPPT Control/1(windSpeed)
  Less than or equal to/1 -> MPPT Control/Enable
  Greater than/1 -> Derating Control/Enable
  MPPT Control/1(activePowerDemand) -> Limiter Function Power Demand/1(activePowerDemandMPPT)
  Derating Control/1(activePowerDemand) -> Limiter Function Power Demand/2(activePowerDemandDerating)
  Limiter Function Power Demand/1(activePowerDemand) -> activePowerDemand/1

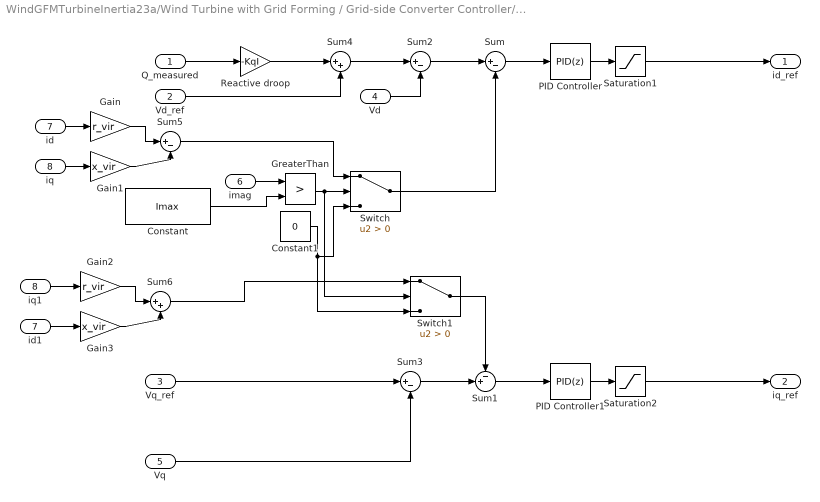
== system WindGFMTurbineInertia23a/Wind Turbine with Grid Forming / Grid-side Converter Controller/Current Reference Generator ==
  Q_measured : Inport
  Vd_ref : Inport  Port=2
  Vq_ref : Inport  Port=3
  Vd : Inport  Port=4
  Vq : Inport  Port=5
  imag : Inport  Port=6
  id : Inport  Port=7
  iq : Inport  Port=8
  Constant : Constant  Value=Imax
  Constant1 : Constant  Value=0
  Gain : Gain  Gain=r_vir
  Gain1 : Gain  Gain=x_vir
  Gain2 : Gain  Gain=r_vir
  Gain3 : Gain  Gain=x_vir
  GreaterThan : RelationalOperator  Operator=>  OutDataTypeStr=boolean  RndMeth=Simplest  InputSameDT=off
  PID Controller : slpidlib/PID Controller  Controller=PID  Form=Parallel  TimeDomain=Discrete-time  UseExternalTs=off  SampleTime=-1  IntegratorMethod=Forward Euler  FilterMethod=Forward Euler  ControllerParametersSource=internal  P=0.9  I=0.5  UseKiTs=off  D=windController.kdvgfm  N=100  UseFilter=on  TunerSelectOption=Transfer Function Based (PID Tuner App)  InitialConditionSource=internal  InitialConditionForIntegrator=0  InitialConditionForFilter=0  DifferentiatorICPrevScaledInput=0  ExternalReset=none  TrackingMode=off  Kt=1  LimitOutput=off  SatLimitsSource=internal  UpperSaturationLimit=Imax/sqrt(2)  LowerSaturationLimit=-Imax/sqrt(2)  LinearizeAsGain=off  AntiWindupMode=back-calculation  Kb=1  LimitIntegrator=off  UpperIntegratorSaturationLimit=inf  LowerIntegratorSaturationLimit=-inf  POutMin=[]  POutMax=[]  IOutMin=[]  IOutMax=[]  DOutMin=[]  DOutMax=[]  NOutMin=[]  NOutMax=[]  SumOutMin=[]  SumOutMax=[]  SaturationOutMin=[]  SaturationOutMax=[]  PParamMin=[]  PParamMax=[]  IParamMin=[]  IParamMax=[]  DParamMin=[]  DParamMax=[]  NParamMin=[]  NParamMax=[]  KbParamMin=[]  KbParamMax=[]  KtParamMin=[]  KtParamMax=[]  KbOutMin=[]  KbOutMax=[]  KtOutMin=[]  KtOutMax=[]  IntegratorOutMin=[]  IntegratorOutMax=[]  FilterOutMin=[]  FilterOutMax=[]  SumI1OutMin=[]  SumI1OutMax=[]  SumI2OutMin=[]  SumI2OutMax=[]  SumI3OutMin=[]  SumI3OutMax=[]  SumI4OutMin=[]  SumI4OutMax=[]  SumDOutMin=[]  SumDOutMax=[]  DifferentiatorOutMin=[]  DifferentiatorOutMax=[]  FilterDiffOutCoefMin=[]  FilterDiffOutCoefMax=[]  ReciprocalOutMin=[]  ReciprocalOutMax=[]  SumDenOutMin=[]  SumDenOutMax=[]  SumNumOutMin=[]  SumNumOutMax=[]  DivideOutMin=[]  DivideOutMax=[]  UdiffTsProdOutMin=[]  UdiffTsProdOutMax=[]  NTsProdOutMin=[]  NTsProdOutMax=[]  UintegralTsProdOutMin=[]  UintegralTsProdOutMax=[]  UngainTsProdOutMin=[]  UngainTsProdOutMax=[]  ClampingZeroOutDataTypeStr=Inherit: Inherit via back propagation  ClampingZeroOutMin=[]  ClampingZeroOutMax=[]  FilterDenConstantOutDataTypeStr=Inherit: Inherit via back propagation  FilterDenConstantOutMin=[]  FilterDenConstantOutMax=[]  PCopyOutDataTypeStr=Inherit: Inherit via back propagation  PCopyOutMin=[]  PCopyOutMax=[]  NCopyOutDataTypeStr=Inherit: Inherit via back propagation  NCopyOutMin=[]  NCopyOutMax=[]  IntegratorContinuousStateAttributes=''  IntegratorStateMustResolveToSignalObject=off  IntegratorRTWStateStorageClass=Auto  FilterContinuousStateAttributes=''  FilterStateMustResolveToSignalObject=off  FilterRTWStateStorageClass=Auto  ParallelPVariant=InternalParameters  IdealPVariant=Disabled  IVariant=InternalParameters  DVariant=InternalParameters  IntegratorVariant=Discrete  SatVariant=Disabled  AWVariant=Passthrough  PCopyVariant=Disabled  TRVariant=Disabled  FdbkBlocksVariant=Forward  IdealPFdbkVariant=Disabled  SatFdbkVariant=Disabled  DerivativeFilterVariant=ForwardEulerFilter  NVariant=InternalParameters  NCopyVariant=Disabled  FilterICVariant=InternalICsFilter  IntegratorICVariant=InternalICs  ExternalResetVariant=Disabled  TRSumVariant=Passthrough  SumFdbkVariant=Disabled  SumVariant=Sum_PID  TsampFilterVariant=InternalTs  TsampNgainVariant=Passthrough  TsampIntegralVariant=Disabled_SignalSpec  ExternalSaturationOutDataTypeStr=Inherit: Same as second input
  PID Controller1 : slpidlib/PID Controller  Controller=PID  Form=Parallel  TimeDomain=Discrete-time  UseExternalTs=off  SampleTime=-1  IntegratorMethod=Forward Euler  FilterMethod=Forward Euler  ControllerParametersSource=internal  P=0.9  I=0.5  UseKiTs=off  D=windController.kdvgfm  N=100  UseFilter=on  TunerSelectOption=Transfer Function Based (PID Tuner App)  InitialConditionSource=internal  InitialConditionForIntegrator=0  InitialConditionForFilter=0  DifferentiatorICPrevScaledInput=0  ExternalReset=none  TrackingMode=off  Kt=1  LimitOutput=off  SatLimitsSource=internal  UpperSaturationLimit=Imax/sqrt(2)  LowerSaturationLimit=-Imax/sqrt(2)  LinearizeAsGain=on  AntiWindupMode=back-calculation  Kb=1  LimitIntegrator=off  UpperIntegratorSaturationLimit=inf  LowerIntegratorSaturationLimit=-inf  POutMin=[]  POutMax=[]  IOutMin=[]  IOutMax=[]  DOutMin=[]  DOutMax=[]  NOutMin=[]  NOutMax=[]  SumOutMin=[]  SumOutMax=[]  SaturationOutMin=[]  SaturationOutMax=[]  PParamMin=[]  PParamMax=[]  IParamMin=[]  IParamMax=[]  DParamMin=[]  DParamMax=[]  NParamMin=[]  NParamMax=[]  KbParamMin=[]  KbParamMax=[]  KtParamMin=[]  KtParamMax=[]  KbOutMin=[]  KbOutMax=[]  KtOutMin=[]  KtOutMax=[]  IntegratorOutMin=[]  IntegratorOutMax=[]  FilterOutMin=[]  FilterOutMax=[]  SumI1OutMin=[]  SumI1OutMax=[]  SumI2OutMin=[]  SumI2OutMax=[]  SumI3OutMin=[]  SumI3OutMax=[]  SumI4OutMin=[]  SumI4OutMax=[]  SumDOutMin=[]  SumDOutMax=[]  DifferentiatorOutMin=[]  DifferentiatorOutMax=[]  FilterDiffOutCoefMin=[]  FilterDiffOutCoefMax=[]  ReciprocalOutMin=[]  ReciprocalOutMax=[]  SumDenOutMin=[]  SumDenOutMax=[]  SumNumOutMin=[]  SumNumOutMax=[]  DivideOutMin=[]  DivideOutMax=[]  UdiffTsProdOutMin=[]  UdiffTsProdOutMax=[]  NTsProdOutMin=[]  NTsProdOutMax=[]  UintegralTsProdOutMin=[]  UintegralTsProdOutMax=[]  UngainTsProdOutMin=[]  UngainTsProdOutMax=[]  ClampingZeroOutDataTypeStr=Inherit: Inherit via back propagation  ClampingZeroOutMin=[]  ClampingZeroOutMax=[]  FilterDenConstantOutDataTypeStr=Inherit: Inherit via back propagation  FilterDenConstantOutMin=[]  FilterDenConstantOutMax=[]  PCopyOutDataTypeStr=Inherit: Inherit via back propagation  PCopyOutMin=[]  PCopyOutMax=[]  NCopyOutDataTypeStr=Inherit: Inherit via back propagation  NCopyOutMin=[]  NCopyOutMax=[]  IntegratorContinuousStateAttributes=''  IntegratorStateMustResolveToSignalObject=off  IntegratorRTWStateStorageClass=Auto  FilterContinuousStateAttributes=''  FilterStateMustResolveToSignalObject=off  FilterRTWStateStorageClass=Auto  ParallelPVariant=InternalParameters  IdealPVariant=Disabled  IVariant=InternalParameters  DVariant=InternalParameters  IntegratorVariant=Discrete  SatVariant=Disabled  AWVariant=Passthrough  PCopyVariant=Disabled  TRVariant=Disabled  FdbkBlocksVariant=Forward  IdealPFdbkVariant=Disabled  SatFdbkVariant=Disabled  DerivativeFilterVariant=ForwardEulerFilter  NVariant=InternalParameters  NCopyVariant=Disabled  FilterICVariant=InternalICsFilter  IntegratorICVariant=InternalICs  ExternalResetVariant=Disabled  TRSumVariant=Passthrough  SumFdbkVariant=Disabled  SumVariant=Sum_PID  TsampFilterVariant=InternalTs  TsampNgainVariant=Passthrough  TsampIntegralVariant=Disabled_SignalSpec  ExternalSaturationOutDataTypeStr=Inherit: Same as second input
  Reactive droop : Gain  Gain=-KqI
  Saturation1 : Saturate  UpperLimit=Imax/sqrt(2)  LowerLimit=-Imax/sqrt(2)
  Saturation2 : Saturate  UpperLimit=Imax/sqrt(2)  LowerLimit=-Imax/sqrt(2)
  Sum{,2..3,5} (4 alike) : Sum  Inputs=|+-
  Sum1 : Sum  Inputs=-+|
  Sum4 : Sum  Inputs=|++
  Sum6 : Sum  Inputs=|++
  Switch : Switch  Criteria=u2 > Threshold  SaturateOnIntegerOverflow=off  InputSameDT=off
  Switch1 : Switch  Criteria=u2 > Threshold  SaturateOnIntegerOverflow=off  InputSameDT=off
  id1 : InportShadow  Port=7
  iq1 : InportShadow  Port=8
  id_ref : Outport
  iq_ref : Outport  Port=2
  wires:
  Switch1/1 -> Sum1/1
  Switch/1 -> Sum/2
  Sum1/1 -> PID Controller1/1
  Sum6/1 -> Switch1/1
  Gain2/1 -> Sum6/1
  iq1/1 -> Gain2/1
  Gain3/1 -> Sum6/2
  id1/1 -> Gain3/1
  Sum5/1 -> Switch/1
  Gain1/1 -> Sum5/2
  Gain/1 -> Sum5/1
  iq/1 -> Gain1/1
  id/1 -> Gain/1
  Constant1/1 -> Switch/3, Switch1/3
  GreaterThan/1 -> Switch1/2, Switch/2
  Sum3/1 -> Sum1/2
  Sum2/1 -> Sum/1
  Sum/1 -> PID Controller/1
  imag/1 -> GreaterThan/1
  Vd_ref/1 -> Sum4/2
  Vq/1 -> Sum3/2
  Vq_ref/1 -> Sum3/1
  Vd/1 -> Sum2/2
  Sum4/1 -> Sum2/1
  Q_measured/1 -> Reactive droop/1
  Reactive droop/1 -> Sum4/1
  PID Controller/1 -> Saturation1/1
  PID Controller1/1 -> Saturation2/1
  Saturation1/1 -> id_ref/1
  Saturation2/1 -> iq_ref/1
  Constant/1 -> GreaterThan/2

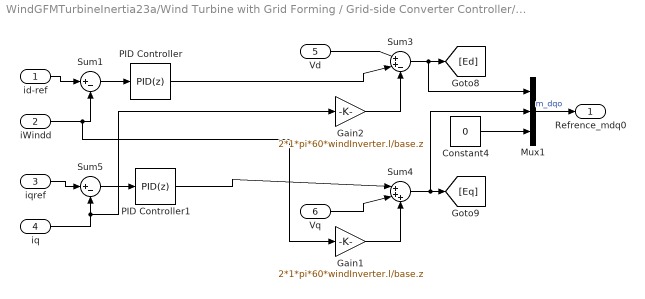
== system WindGFMTurbineInertia23a/Wind Turbine with Grid Forming / Grid-side Converter Controller/Current_controller ==
  id-ref : Inport
  iWindd : Inport  Port=2
  iqref : Inport  Port=3
  iq : Inport  Port=4
  Vd : Inport  Port=5
  Vq : Inport  Port=6
  Constant4 : Constant  Value=0
  Gain1 : Gain  Gain=2*1*pi*60*windInverter.l/base.z
  Gain2 : Gain  Gain=2*1*pi*60*windInverter.l/base.z
  Mux1 : Mux  Inputs=3
  PID Controller : slpidlib/PID Controller  Controller=PID  Form=Parallel  TimeDomain=Discrete-time  UseExternalTs=off  SampleTime=-1  IntegratorMethod=Forward Euler  FilterMethod=Forward Euler  ControllerParametersSource=internal  P=windController.kpic  I=windController.kiic  UseKiTs=off  D=windController.kd  N=100  UseFilter=on  TunerSelectOption=Transfer Function Based (PID Tuner App)  InitialConditionSource=internal  InitialConditionForIntegrator=0  InitialConditionForFilter=0  DifferentiatorICPrevScaledInput=0  ExternalReset=none  TrackingMode=off  Kt=1  LimitOutput=off  SatLimitsSource=internal  UpperSaturationLimit=inf  LowerSaturationLimit=-inf  LinearizeAsGain=on  AntiWindupMode=none  Kb=1  LimitIntegrator=off  UpperIntegratorSaturationLimit=inf  LowerIntegratorSaturationLimit=-inf  POutMin=[]  POutMax=[]  IOutMin=[]  IOutMax=[]  DOutMin=[]  DOutMax=[]  NOutMin=[]  NOutMax=[]  SumOutMin=[]  SumOutMax=[]  SaturationOutMin=[]  SaturationOutMax=[]  PParamMin=[]  PParamMax=[]  IParamMin=[]  IParamMax=[]  DParamMin=[]  DParamMax=[]  NParamMin=[]  NParamMax=[]  KbParamMin=[]  KbParamMax=[]  KtParamMin=[]  KtParamMax=[]  KbOutMin=[]  KbOutMax=[]  KtOutMin=[]  KtOutMax=[]  IntegratorOutMin=[]  IntegratorOutMax=[]  FilterOutMin=[]  FilterOutMax=[]  SumI1OutMin=[]  SumI1OutMax=[]  SumI2OutMin=[]  SumI2OutMax=[]  SumI3OutMin=[]  SumI3OutMax=[]  SumI4OutMin=[]  SumI4OutMax=[]  SumDOutMin=[]  SumDOutMax=[]  DifferentiatorOutMin=[]  DifferentiatorOutMax=[]  FilterDiffOutCoefMin=[]  FilterDiffOutCoefMax=[]  ReciprocalOutMin=[]  ReciprocalOutMax=[]  SumDenOutMin=[]  SumDenOutMax=[]  SumNumOutMin=[]  SumNumOutMax=[]  DivideOutMin=[]  DivideOutMax=[]  UdiffTsProdOutMin=[]  UdiffTsProdOutMax=[]  NTsProdOutMin=[]  NTsProdOutMax=[]  UintegralTsProdOutMin=[]  UintegralTsProdOutMax=[]  UngainTsProdOutMin=[]  UngainTsProdOutMax=[]  ClampingZeroOutDataTypeStr=Inherit: Inherit via back propagation  ClampingZeroOutMin=[]  ClampingZeroOutMax=[]  FilterDenConstantOutDataTypeStr=Inherit: Inherit via back propagation  FilterDenConstantOutMin=[]  FilterDenConstantOutMax=[]  PCopyOutDataTypeStr=Inherit: Inherit via back propagation  PCopyOutMin=[]  PCopyOutMax=[]  NCopyOutDataTypeStr=Inherit: Inherit via back propagation  NCopyOutMin=[]  NCopyOutMax=[]  IntegratorContinuousStateAttributes=''  IntegratorStateMustResolveToSignalObject=off  IntegratorRTWStateStorageClass=Auto  FilterContinuousStateAttributes=''  FilterStateMustResolveToSignalObject=off  FilterRTWStateStorageClass=Auto  ParallelPVariant=InternalParameters  IdealPVariant=Disabled  IVariant=InternalParameters  DVariant=InternalParameters  IntegratorVariant=Discrete  SatVariant=Disabled  AWVariant=Passthrough  PCopyVariant=Disabled  TRVariant=Disabled  FdbkBlocksVariant=Forward  IdealPFdbkVariant=Disabled  SatFdbkVariant=Disabled  DerivativeFilterVariant=ForwardEulerFilter  NVariant=InternalParameters  NCopyVariant=Disabled  FilterICVariant=InternalICsFilter  IntegratorICVariant=InternalICs  ExternalResetVariant=Disabled  TRSumVariant=Passthrough  SumFdbkVariant=Disabled  SumVariant=Sum_PID  TsampFilterVariant=InternalTs  TsampNgainVariant=Passthrough  TsampIntegralVariant=Disabled_SignalSpec  ExternalSaturationOutDataTypeStr=Inherit: Same as second input
  PID Controller1 : slpidlib/PID Controller  Controller=PID  Form=Parallel  TimeDomain=Discrete-time  UseExternalTs=off  SampleTime=-1  IntegratorMethod=Forward Euler  FilterMethod=Forward Euler  ControllerParametersSource=internal  P=windController.kpic  I=windController.kiic  UseKiTs=off  D=windController.kd  N=100  UseFilter=on  TunerSelectOption=Transfer Function Based (PID Tuner App)  InitialConditionSource=internal  InitialConditionForIntegrator=0  InitialConditionForFilter=0  DifferentiatorICPrevScaledInput=0  ExternalReset=none  TrackingMode=off  Kt=1  LimitOutput=off  SatLimitsSource=internal  UpperSaturationLimit=inf  LowerSaturationLimit=-inf  LinearizeAsGain=on  AntiWindupMode=none  Kb=1  LimitIntegrator=off  UpperIntegratorSaturationLimit=inf  LowerIntegratorSaturationLimit=-inf  POutMin=[]  POutMax=[]  IOutMin=[]  IOutMax=[]  DOutMin=[]  DOutMax=[]  NOutMin=[]  NOutMax=[]  SumOutMin=[]  SumOutMax=[]  SaturationOutMin=[]  SaturationOutMax=[]  PParamMin=[]  PParamMax=[]  IParamMin=[]  IParamMax=[]  DParamMin=[]  DParamMax=[]  NParamMin=[]  NParamMax=[]  KbParamMin=[]  KbParamMax=[]  KtParamMin=[]  KtParamMax=[]  KbOutMin=[]  KbOutMax=[]  KtOutMin=[]  KtOutMax=[]  IntegratorOutMin=[]  IntegratorOutMax=[]  FilterOutMin=[]  FilterOutMax=[]  SumI1OutMin=[]  SumI1OutMax=[]  SumI2OutMin=[]  SumI2OutMax=[]  SumI3OutMin=[]  SumI3OutMax=[]  SumI4OutMin=[]  SumI4OutMax=[]  SumDOutMin=[]  SumDOutMax=[]  DifferentiatorOutMin=[]  DifferentiatorOutMax=[]  FilterDiffOutCoefMin=[]  FilterDiffOutCoefMax=[]  ReciprocalOutMin=[]  ReciprocalOutMax=[]  SumDenOutMin=[]  SumDenOutMax=[]  SumNumOutMin=[]  SumNumOutMax=[]  DivideOutMin=[]  DivideOutMax=[]  UdiffTsProdOutMin=[]  UdiffTsProdOutMax=[]  NTsProdOutMin=[]  NTsProdOutMax=[]  UintegralTsProdOutMin=[]  UintegralTsProdOutMax=[]  UngainTsProdOutMin=[]  UngainTsProdOutMax=[]  ClampingZeroOutDataTypeStr=Inherit: Inherit via back propagation  ClampingZeroOutMin=[]  ClampingZeroOutMax=[]  FilterDenConstantOutDataTypeStr=Inherit: Inherit via back propagation  FilterDenConstantOutMin=[]  FilterDenConstantOutMax=[]  PCopyOutDataTypeStr=Inherit: Inherit via back propagation  PCopyOutMin=[]  PCopyOutMax=[]  NCopyOutDataTypeStr=Inherit: Inherit via back propagation  NCopyOutMin=[]  NCopyOutMax=[]  IntegratorContinuousStateAttributes=''  IntegratorStateMustResolveToSignalObject=off  IntegratorRTWStateStorageClass=Auto  FilterContinuousStateAttributes=''  FilterStateMustResolveToSignalObject=off  FilterRTWStateStorageClass=Auto  ParallelPVariant=InternalParameters  IdealPVariant=Disabled  IVariant=InternalParameters  DVariant=InternalParameters  IntegratorVariant=Discrete  SatVariant=Disabled  AWVariant=Passthrough  PCopyVariant=Disabled  TRVariant=Disabled  FdbkBlocksVariant=Forward  IdealPFdbkVariant=Disabled  SatFdbkVariant=Disabled  DerivativeFilterVariant=ForwardEulerFilter  NVariant=InternalParameters  NCopyVariant=Disabled  FilterICVariant=InternalICsFilter  IntegratorICVariant=InternalICs  ExternalResetVariant=Disabled  TRSumVariant=Passthrough  SumFdbkVariant=Disabled  SumVariant=Sum_PID  TsampFilterVariant=InternalTs  TsampNgainVariant=Passthrough  TsampIntegralVariant=Disabled_SignalSpec  ExternalSaturationOutDataTypeStr=Inherit: Same as second input
  Sum1 : Sum  Inputs=|+-
  Sum3 : Sum  Inputs=|++-
  Sum4 : Sum  Inputs=|+++
  Sum5 : Sum  Inputs=|+-
  Refrence_mdq0 : Outport
  wires:
  PID Controller/1 -> Sum3/2
  Sum3/1 -> Mux1/1, [Ed]
  Gain2/1 -> Sum3/3
  iWindd/1 -> Gain1/1, Sum1/2
  id-ref/1 -> Sum1/1
  Gain1/1 -> Sum4/3
  Vq/1 -> Sum4/2
  iq/1 -> Gain2/1, Sum5/2
  Sum1/1 -> PID Controller/1
  Vd/1 -> Sum3/1
  Constant4/1 -> Mux1/3
  Sum5/1 -> PID Controller1/1
  iqref/1 -> Sum5/1
  PID Controller1/1 -> Sum4/1
  Sum4/1 -> Mux1/2, [Eq]
  Mux1/1 -> Refrence_mdq0/1  "m_dqo"

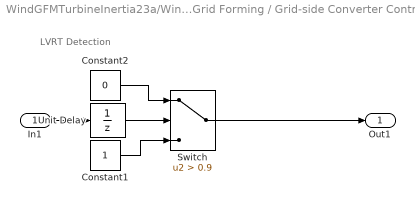
== system WindGFMTurbineInertia23a/Wind Turbine with Grid Forming / Grid-side Converter Controller/DC Bus Chopper control  ==
  note: LVRT Detection
  In1 : Inport
  Constant1 : Constant
  Constant2 : Constant  Value=0
  Switch : Switch  Criteria=u2 > Threshold  Threshold=0.9  SaturateOnIntegerOverflow=off  InputSameDT=off
  Unit Delay : UnitDelay  SampleTime=-1  HasFrameUpgradeWarning=on
  Out1 : Outport
  wires:
  Unit Delay/1 -> Switch/2
  In1/1 -> Unit Delay/1
  Constant2/1 -> Switch/1
  Constant1/1 -> Switch/3
  Switch/1 -> Out1/1

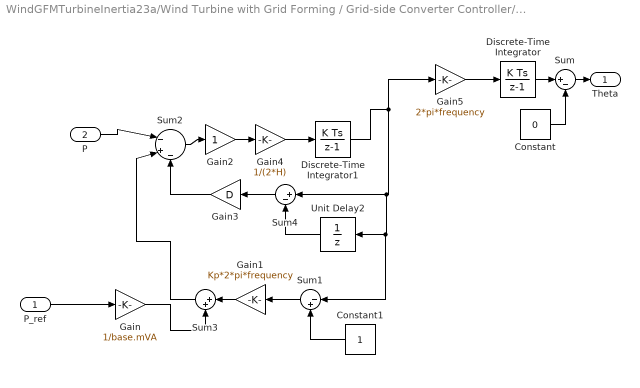
== system WindGFMTurbineInertia23a/Wind Turbine with Grid Forming / Grid-side Converter Controller/Grid Forming Reference Generator ==
  P_ref : Inport
  P : Inport  Port=2
  Constant : Constant  Value=0
  Constant1 : Constant
  Discrete-Time Integrator : DiscreteIntegrator  SampleTime=Ts  ICPrevOutput=DiscIntNeverNeededParam  ICPrevScaledInput=DiscIntNeverNeededParam
  Discrete-Time Integrator1 : DiscreteIntegrator  InitialCondition=0.99  SampleTime=Ts  ICPrevOutput=DiscIntNeverNeededParam  ICPrevScaledInput=DiscIntNeverNeededParam
  Gain : Gain  Gain=1/base.mVA
  Gain1 : Gain  Gain=Kp*2*pi*frequency
  Gain2 : Gain
  Gain3 : Gain  Gain=D
  Gain4 : Gain  Gain=1/(2*H)
  Gain5 : Gain  Gain=2*pi*frequency
  Sum : Sum  Inputs=|+-
  Sum1 : Sum  Inputs=|-+
  Sum2 : Sum  Inputs=|-+-
  Sum3 : Sum  Inputs=|++
  Sum4 : Sum  Inputs=|+-
  Unit Delay2 : UnitDelay  SampleTime=-1  HasFrameUpgradeWarning=on
  Theta : Outport
  wires:
  Sum3/1 -> Sum2/2
  Gain/1 -> Sum3/2
  Gain1/1 -> Sum3/1
  Discrete-Time Integrator1/1 -> Sum4/1, Unit Delay2/1, Sum1/1, Gain5/1
  Sum1/1 -> Gain1/1
  Constant1/1 -> Sum1/2
  Constant/1 -> Sum/2
  Sum/1 -> Theta/1
  Discrete-Time Integrator/1 -> Sum/1
  Gain5/1 -> Discrete-Time Integrator/1
  Gain2/1 -> Gain4/1
  Sum2/1 -> Gain2/1
  P/1 -> Sum2/1
  Unit Delay2/1 -> Sum4/2
  Sum4/1 -> Gain3/1
  Gain3/1 -> Sum2/3
  Gain4/1 -> Discrete-Time Integrator1/1
  P_ref/1 -> Gain/1
